simulink model "kalmanfilter"  (R2015a)
settings: Solver=FixedStepDiscrete  StartTime=0.0  StopTime=10.0  RelTol=1e-3
values from neighbouring files (symbols this model uses):
  Q = 0.00001    (= 1e-05)    [kalmanTest.m]
  R = 0.001    [kalmanTest.m]
undefined symbols (not defined in the file or in its folder): A, B, C, D, x0
undefined symbols (not defined in the file): A1, B1, C1, D1, P1, Q1, R1, x1
settings Model: Creator=fo1521  LastModifiedBy=jinkale
settings DataIOCC: SignalLoggingSaveFormat=ModelDataLogs
settings OptimizationCC: ExpressionDepthLimit=2147483647  InitFltsAndDblsToZero=on
settings DebuggingCC: SaveWithParameterizedLinksMsg=none  UnderspecifiedInitializationDetection=Classic  MergeDetectMultiDrivingBlocksExec=none  SolverPrmCheckMsg=warning  MultiTaskCondExecSysMsg=none  FcnCallInpInsideContextMsg=UseLocalSettings  StateNameClashWarn=warning  StrictBusMsg=None
settings HardwareCC: TargetHWDeviceType=32-bit Generic
settings GRTTargetCC: TargetFcnLib=ansi_tfl_tmw.mat  CombineOutputUpdateFcns=off  GRTInterface=on

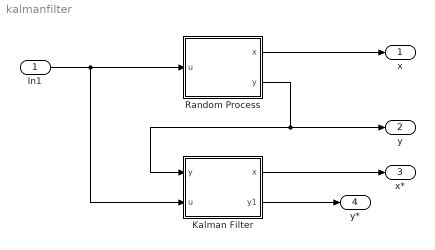
== system kalmanfilter ==
  In1 : Inport
  Kalman Filter : Subsystem  mask{x0=x1, P0=P1, A=A1, B=B1, C=C1, D=D1, Q=Q1, R=R1}
      mask help:
      | Linear Random Process
      | x(k+1)=Ax(k)+Bu(k)+w
      | y(k)=Cx(k)+Du(k)+v
      | w~N(0,Q)
      | w~N(0,R)
      mask Display:
      | disp(sprintf('Kalman\n Filter'))
      | port_label('output',2,'y')
      | port_label('output',1,'x')
      | port_label('input',1,'y')
      | port_label('input',2,'u')
  Random Process : Subsystem  mask{x0=x0, A=A, B=B, C=C, D=D, Q=sqrt(Q), R=sqrt(R)}
      mask help:
      | Linear Random Process
      | x(k+1)=Ax(k)+Bu(k)+w
      | y(k)=Cx(k)+Du(k)+v
      | w~N(0,Q)
      | w~N(0,R)
      mask Display:
      | disp(sprintf('Linear\n Random\n System'))
      | port_label('output',1,'x')
      | port_label('output',2,'y')
      | port_label('input',1,'u')
  x : Outport
  y : Outport  Port=2
  x* : Outport  Port=3
  y* : Outport  Port=4
  wires:
  Random Process/2(y) -> Kalman Filter/1(y), y/1
  In1/1 -> Random Process/1(u), Kalman Filter/2(u)
  Random Process/1(x) -> x/1
  Kalman Filter/1(x) -> x*/1
  Kalman Filter/2(y1) -> y*/1

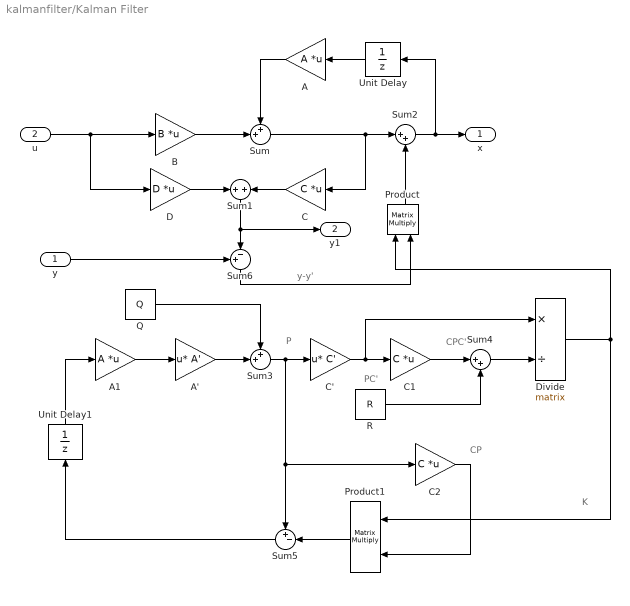
== system kalmanfilter/Kalman Filter ==
  note: P
  note: PC'
  note: CPC'
  note: K
  note: CP
  note: y-y'
  y : Inport
  u : Inport  Port=2  PortDimensions=size(B,2)
  A : Gain  Gain=A  Multiplication=Matrix(K*u)
  A' : Gain  Gain=A'  Multiplication=Matrix(u*K)
  A1 : Gain  Gain=A  Multiplication=Matrix(K*u)
  B : Gain  Gain=B  Multiplication=Matrix(K*u)
  C : Gain  Gain=C  Multiplication=Matrix(K*u)
  C' : Gain  Gain=C'  Multiplication=Matrix(u*K)
  C1 : Gain  Gain=C  Multiplication=Matrix(K*u)
  C2 : Gain  Gain=C  Multiplication=Matrix(K*u)
  D : Gain  Gain=D  Multiplication=Matrix(K*u)
  Divide : Product  Inputs=*/  Multiplication=Matrix(*)
  Product : Product  Multiplication=Matrix(*)  RndMeth=Zero
  Product1 : Product  Multiplication=Matrix(*)  RndMeth=Zero
  Q : Constant  Value=Q
  R : Constant  Value=R
  Sum : Sum  Inputs=++|
  Sum1 : Sum  Inputs=+|+
  Sum2 : Sum  Inputs=|++
  Sum3 : Sum  Inputs=++|
  Sum4 : Sum  Inputs=|++
  Sum5 : Sum  Inputs=+-|
  Sum6 : Sum  Inputs=+-|
  Unit Delay : UnitDelay  InitialCondition=x0
  Unit Delay1 : UnitDelay  InitialCondition=P0
  x : Outport
  y1 : Outport  Port=2
  wires:
  u/1 -> B/1, D/1
  B/1 -> Sum/2
  A/1 -> Sum/1
  Unit Delay/1 -> A/1
  Sum/1 -> Sum2/1, C/1
  Sum2/1 -> x/1, Unit Delay/1
  D/1 -> Sum1/1
  C/1 -> Sum1/2
  A1/1 -> A'/1
  A'/1 -> Sum3/2
  Q/1 -> Sum3/1
  Sum3/1 -> C'/1, Sum5/1, C2/1
  C'/1 -> C1/1, Divide/1
  Product/1 -> Sum2/2
  Divide/1 -> Product/1, Product1/1
  Product1/1 -> Sum5/2
  C1/1 -> Sum4/1
  R/1 -> Sum4/2
  Sum4/1 -> Divide/2
  Unit Delay1/1 -> A1/1
  Sum5/1 -> Unit Delay1/1
  C2/1 -> Product1/2
  Sum1/1 -> Sum6/2, y1/1
  y/1 -> Sum6/1
  Sum6/1 -> Product/2

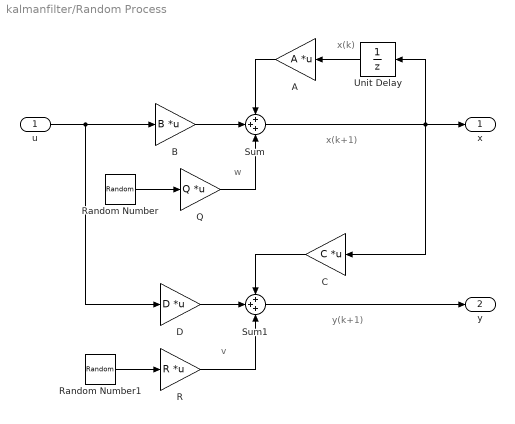
== system kalmanfilter/Random Process ==
  note: x(k+1)
  note: y(k+1)
  note: x(k)
  note: w
  note: v
  u : Inport  PortDimensions=size(B,2)
  A : Gain  Gain=A  Multiplication=Matrix(K*u)
  B : Gain  Gain=B  Multiplication=Matrix(K*u)
  C : Gain  Gain=C  Multiplication=Matrix(K*u)
  D : Gain  Gain=D  Multiplication=Matrix(K*u)
  Q : Gain  Gain=Q  Multiplication=Matrix(K*u)
  R : Gain  Gain=R  Multiplication=Matrix(K*u)
  Random Number : RandomNumber  Mean=zeros(size(Q,1),1)  Variance=ones(size(Q,1),1)  Seed=7  SampleTime=1
  Random Number1 : RandomNumber  Mean=zeros(size(R,1),1)  Variance=ones(size(R,1),1)  SampleTime=1
  Sum : Sum  Inputs=+++
  Sum1 : Sum  Inputs=+++
  Unit Delay : UnitDelay  InitialCondition=x0
  x : Outport
  y : Outport  Port=2
  wires:
  u/1 -> B/1, D/1
  Random Number/1 -> Q/1
  B/1 -> Sum/2
  C/1 -> Sum1/1
  D/1 -> Sum1/2
  Random Number1/1 -> R/1
  R/1 -> Sum1/3
  Sum1/1 -> y/1
  Sum/1 -> Unit Delay/1, x/1, C/1
  Unit Delay/1 -> A/1
  A/1 -> Sum/1
  Q/1 -> Sum/3
